simulink model "own_collector"  (R2018a)
settings: Solver=VariableStepAuto  StartTime=0.0  StopTime=120  FixedStep=0.01  MaxStep=0.01  RelTol=1e-5
libraries: simulink x2
settings Model: Creator=daniel  LastModifiedBy=blond
settings SolverCC: ZeroCrossAlgorithm=Adaptive  AlgebraicLoopSolver=LineSearch
settings DebuggingCC: MaxConsecutiveZCsMsg=warning

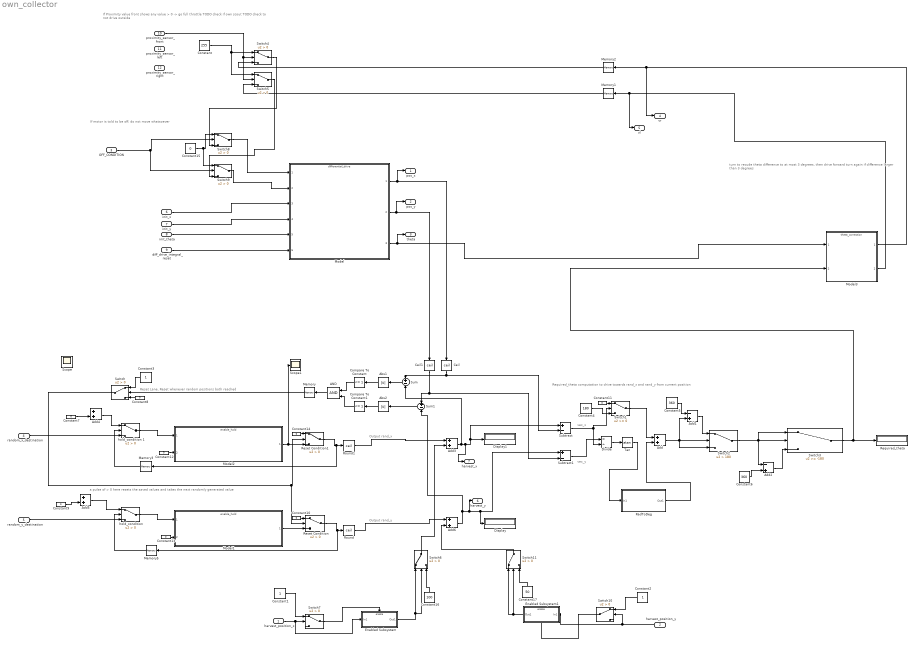
== system own_collector ==
  note: If Proximity value front shows any value > 0  -> go full throttle
      | TODO check if own scout
      | TODO check to not drive outside
  note: If motor is told to be off, do not move whatsoever
  note: turn to recude theta difference to at
      | most 3 degrees, then drive forward
      | turn again if difference larger than
      | 3 degrees
  note: Required_theta computation to drive towards rand_x and rand_y from current position
  note: vec_y
  note: Reset Lane, Reset whenever random positions both reached
  note: a pulse of > 0 here resets the saved values and takes the next randomly generated value
  note: Output rand_x
  note: Output rand_y
  note: vec_x
  harvest_position_x : Inport
  harvest_position_y : Inport  Port=2
  "OFF_CONDITION " : Inport  Port=3
  random_x_destination : Inport  Port=4
  random_y_destination : Inport  Port=5
  "init_x " : Inport  Port=6
  init_y : Inport  Port=7
  "init_theta " : Inport  Port=8
  diff_drive_integral_reset : Inport  Port=9
  proximity_sensor_front : Inport  Port=10
  proximity_sensor_left : Inport  Port=11
  proximity_sensor_right : Inport  Port=12
  AND : Logic  IconShape=distinctive  AllPortsSameDT=off  OutDataTypeStr=boolean
  Abs1 : Abs
  Abs2 : Abs
  Add{,3..6} (5 alike) : Sum
  Add1 : Sum  Inputs=-+
  Add2 : Sum  Inputs=-+
  Ceil : Rounding  Operator=ceil
  Ceil1 : Rounding  Operator=ceil
  Compare To Constant : simulink/Logic and Bit Operations/Compare To Constant  relop=<=  const=1  OutDataTypeStr=boolean
  Compare To Constant1 : simulink/Logic and Bit Operations/Compare To Constant  relop=<=  const=1  OutDataTypeStr=boolean
  Constant : Constant  Value=255
  Constant1 : Constant
  Constant{7..15} (9 alike) : Constant  Value=0
  Constant16 : Constant  Value=100
  Constant17 : Constant  Value=50
  Constant2 : Constant
  Constant3 : Constant
  Constant4 : Constant  Value=180
  Constant5 : Constant  Value=360
  Constant6 : Constant  Value=360
  Display : Display
  Display1 : Display
  Divide : Product  Inputs=*/
  Enabled Subsystem : Subsystem  TreatAsAtomicUnit=on
  Enabled Subsystem1 : Subsystem  TreatAsAtomicUnit=on
  Memory : Memory
  Memory1 : Memory
  Memory2 : Memory
  Memory3 : Memory  InheritSampleTime=on
  Memory5 : Memory  InheritSampleTime=on
  Model : ModelReference  ModelNameDialog=differential_drive.slx  SimulationMode=Normal  ModelReferenceVersion=1.307
  Model1 : ModelReference  ModelNameDialog=enable_hold.slx  SimulationMode=Normal  ModelReferenceVersion=1.282
  Model2 : ModelReference  ModelNameDialog=enable_hold.slx  SimulationMode=Normal  ModelReferenceVersion=1.282
  Model3 : ModelReference  ModelNameDialog=theta_correction.slx  SimulationMode=Normal  ModelReferenceVersion=1.3
  RadToDeg : Subsystem
  Required_theta : Display
  Reset Condition : Switch  Criteria=u2 > Threshold
  Reset Condition1 : Switch  Criteria=u2 > Threshold
  Round : Rounding  Operator=ceil
  Round1 : Rounding  Operator=ceil
  Scope : Scope
  Scope1 : Scope
  Subtract : Sum  Inputs=+-
  Subtract1 : Sum  Inputs=+-
  Sum : Sum  Inputs=+-
  Sum1 : Sum  Inputs=+-
  Switch{,4..11} (9 alike) : Switch  Criteria=u2 > Threshold
  Switch1 : Switch
  Switch2 : Switch  Criteria=u2 > Threshold  Threshold=180
  Switch3 : Switch  Threshold=-180
  Tan : Trigonometry  Operator=atan  OutputSignalType=real
  "hold_condition " : Switch  Criteria=u2 > Threshold
  hold_condition 1 : Switch  Criteria=u2 > Threshold
  pos_x : Outport
  pos_y : Outport  Port=2
  theta : Outport  Port=3
  vr : Outport  Port=4
  vl : Outport  Port=5
  harvest_y : Outport  Port=6
  harvest_x : Outport  Port=7
  wires:
  "init_theta "/1 -> Model/5
  Model/1 -> pos_x/1, Ceil/1
  Model/2 -> pos_y/1, Ceil1/1
  Model/3 -> Model3/1, theta/1
  diff_drive_integral_reset/1 -> Model/6
  "hold_condition "/1 -> Model1/1
  Round/1 -> Add6/1
  Model1/1 -> Reset Condition/3
  Round1/1 -> Add3/1
  Model2/1 -> Scope1/1, Reset Condition1/3
  hold_condition 1/1 -> Model2/1
  Compare To Constant/1 -> AND/1
  Compare To Constant1/1 -> AND/2
  Ceil1/1 -> Sum1/1, Subtract1/2
  Ceil/1 -> Sum/1, Subtract/2
  AND/1 -> Memory/1
  Constant3/1 -> Switch/1
  Memory/1 -> Switch/2
  Switch/1 -> Reset Condition/2, Reset Condition1/2
  Subtract1/1 -> Divide/1
  Subtract/1 -> Switch1/2, Divide/2
  Divide/1 -> Tan/1
  Tan/1 -> RadToDeg/1(In1)
  Switch1/1 -> Add/1
  Constant4/1 -> Switch1/3
  Add/1 -> Switch2/3, Switch2/2, Add1/2
  Constant5/1 -> Add1/1
  Add1/1 -> Switch2/1
  Switch2/1 -> Switch3/1, Switch3/2, Add2/1
  Constant6/1 -> Add2/2
  Add2/1 -> Switch3/3
  Switch3/1 -> Model3/2, Required_theta/1
  RadToDeg/1(Out1) -> Add/2
  Constant7/1 -> Add4/2
  Constant8/1 -> Switch/3
  Constant10/1 -> Reset Condition/1
  Constant11/1 -> Switch1/1
  Constant12/1 -> Model2/2
  Constant13/1 -> Model1/2
  Constant14/1 -> Reset Condition1/1
  Reset Condition1/1 -> Memory3/1, Round1/1
  Reset Condition/1 -> Memory5/1, Round/1
  Sum/1 -> Abs1/1
  Abs1/1 -> Compare To Constant/1
  Abs2/1 -> Compare To Constant1/1
  Sum1/1 -> Abs2/1
  Memory5/1 -> "hold_condition "/2
  Memory3/1 -> hold_condition 1/2
  Add4/1 -> hold_condition 1/1
  Constant9/1 -> Add5/2
  Add5/1 -> "hold_condition "/1
  "OFF_CONDITION "/1 -> Switch9/2, Switch8/2
  Constant15/1 -> Switch9/1, Switch8/1
  Switch8/1 -> Model/1
  Switch9/1 -> Model/2
  "init_x "/1 -> Model/3
  init_y/1 -> Model/4
  Model3/1 -> vr/1, Memory2/1
  Model3/2 -> vl/1, Memory1/1
  proximity_sensor_front/1 -> Switch4/2, Switch5/2
  Constant/1 -> Switch5/1, Switch4/1
  Switch4/1 -> Switch8/3
  Switch5/1 -> Switch9/3
  Memory1/1 -> Switch5/3
  Memory2/1 -> Switch4/3
  harvest_position_y/1 -> Switch10/2, Enabled Subsystem1/1(In1)
  harvest_position_x/1 -> Enabled Subsystem/1(In1), Switch7/2
  Constant1/1 -> Switch7/1
  Switch7/1 -> Enabled Subsystem/Enable
  Constant2/1 -> Switch10/1
  Switch10/1 -> Enabled Subsystem1/Enable
  random_x_destination/1 -> hold_condition 1/3
  random_y_destination/1 -> "hold_condition "/3
  Enabled Subsystem/1(Out1) -> Switch6/2, Switch6/1
  Constant16/1 -> Switch6/3
  Enabled Subsystem1/1(Out1) -> Switch11/2, Switch11/1
  Constant17/1 -> Switch11/3
  Add3/1 -> Sum/2, harvest_x/1, Subtract/1, Display1/1
  Add6/1 -> Sum1/2, harvest_y/1, Display/1, Subtract1/1
  Switch11/1 -> Add6/2
  Switch6/1 -> Add3/2

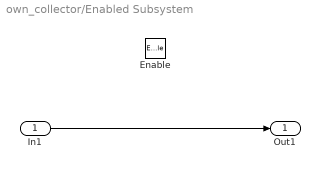
== system own_collector/Enabled Subsystem ==
  In1 : Inport
  Enable : EnablePort
  Out1 : Outport
  wires:
  In1/1 -> Out1/1

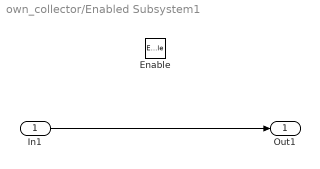
== system own_collector/Enabled Subsystem1 ==
  In1 : Inport
  Enable : EnablePort
  Out1 : Outport
  wires:
  In1/1 -> Out1/1

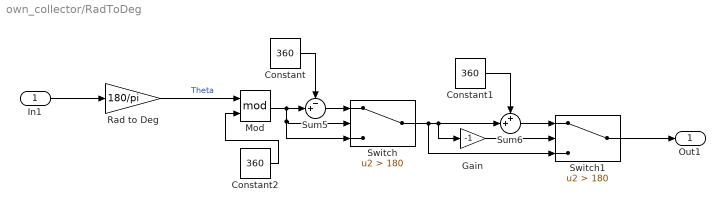
== system own_collector/RadToDeg ==
  In1 : Inport
  Constant : Constant  Value=360
  Constant1 : Constant  Value=360
  Constant2 : Constant  Value=360
  Gain : Gain  Gain=-1
  Mod : Math  Operator=mod  SaturateOnIntegerOverflow=on
  Rad to Deg : Gain  Gain=180/pi
  Sum5 : Sum  Inputs=-+|
  Sum6 : Sum  Inputs=++|
  Switch : Switch  Criteria=u2 > Threshold  Threshold=180
  Switch1 : Switch  Criteria=u2 > Threshold  Threshold=180
  Out1 : Outport
  wires:
  Constant/1 -> Sum5/1
  Constant1/1 -> Sum6/1
  Rad to Deg/1 -> Mod/1  "Theta"
  Gain/1 -> Switch1/2
  Switch/1 -> Sum6/2, Gain/1, Switch1/3
  Sum5/1 -> Switch/1
  Mod/1 -> Sum5/2, Switch/2, Switch/3
  Sum6/1 -> Switch1/1
  Constant2/1 -> Mod/2
  In1/1 -> Rad to Deg/1
  Switch1/1 -> Out1/1
